simulink model "pitch_loop"  (Simulink 9.1)
settings: Solver=VariableStepAuto  StartTime=0.0  StopTime=10  RelTol=1e-3
values from neighbouring files (symbols this model uses):
  G = P.G    [getTF.m]
libraries: cstblocks x1
settings Model: LogicAnalyzerSignalOrdering=e66c3e0b-e53f-4c76-9941-291a87f7b6fd,76aed07c-1e48-440e-8e95-e8f535cd91f0,cd2aeb39-80bf-4c24-8e01-c28722cb3c59  Creator=leonardopedroso  LastModifiedBy=João Pinto
settings DataIOCC: SaveFormat=Dataset
settings OptimizationCC: LifeSpan=auto
settings DebuggingCC: UnderspecifiedInitializationDetection=Simplified  MergeDetectMultiDrivingBlocksExec=error  SFUnexpectedBacktrackingDiag=error  SFNoUnconditionalDefaultTransitionDiag=error  SFExecutionAtInitializationDiag=warning
settings HardwareCC: ProdBitPerPointer=64  ProdBitPerSizeT=64  ProdBitPerPtrDiffT=64  ProdLargestAtomicFloat=Float  ProdIntDivRoundTo=Zero  ProdEndianess=LittleEndian  ProdWordSize=64  ProdHWDeviceType=Intel->x86-64 (Windows64)
settings ModelReferenceCC: PropagateSignalLabelsOutOfModel=on
settings CodeAppCC: StateflowObjectComments=off
settings GRTTargetCC: TargetLangStandard=C99 (ISO)  CombineOutputUpdateFcns=on  GRTInterface=off
settings ConfigComp: CovMetricSettings=dwe  CovHtmlReporting=off  CovSaveCumulativeToWorkspaceVar=off  CovSaveSingleToWorkspaceVar=off  CovExternalEMLEnable=on

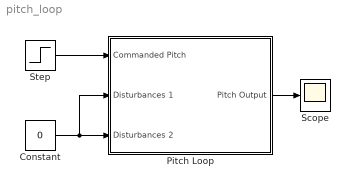
== system pitch_loop ==
  Constant : Constant  Value=0
  "Pitch Loop " : Subsystem
  Scope : Scope
  Step : Step  After=pi/9  SampleTime=0
  wires:
  Constant/1 -> "Pitch Loop "/2(Disturbances 1), "Pitch Loop "/3("Disturbances 2 ")
  "Pitch Loop "/1(Pitch Output) -> Scope/1
  Step/1 -> "Pitch Loop "/1(Commanded Pitch)

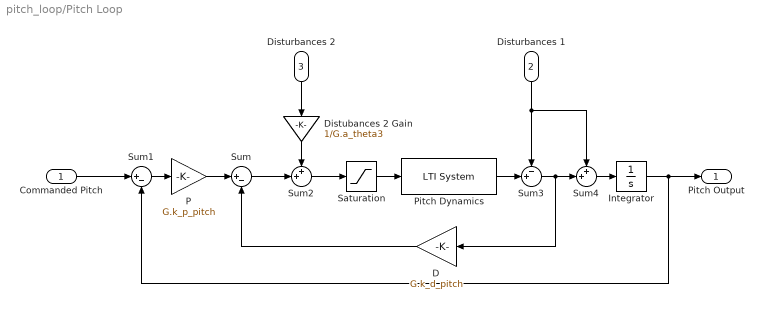
== system pitch_loop/Pitch Loop  ==
  Commanded Pitch : Inport
  Disturbances 1 : Inport  Port=2
  "Disturbances 2 " : Inport  Port=3
  D : Gain  Gain=G.k_d_pitch
  Distubances 2 Gain : Gain  Gain=1/G.a_theta3
  Integrator : Integrator
  "P " : Gain  Gain=G.k_p_pitch
  Pitch Dynamics : cstblocks/LTI System  sys=T_theta_dot_delta_e  IC=[]
  Saturation : Saturate  UpperLimit=G.delta_e_max  LowerLimit=-G.delta_a_max
  Sum : Sum  Inputs=|+-
  Sum1 : Sum  Inputs=|+-
  Sum2 : Sum  Inputs=++|
  Sum3 : Sum  Inputs=-+|
  Sum4 : Sum  Inputs=++|
  Pitch Output : Outport
  wires:
  Integrator/1 -> Pitch Output/1, Sum1/2
  Sum1/1 -> "P "/1
  Sum/1 -> Sum2/2
  Distubances 2 Gain/1 -> Sum2/1
  "Disturbances 2 "/1 -> Distubances 2 Gain/1
  Saturation/1 -> Pitch Dynamics/1
  "P "/1 -> Sum/1
  D/1 -> Sum/2
  Pitch Dynamics/1 -> Sum3/2
  Disturbances 1/1 -> Sum4/1, Sum3/1
  Sum3/1 -> D/1, Sum4/2
  Sum4/1 -> Integrator/1
  Sum2/1 -> Saturation/1
  Commanded Pitch/1 -> Sum1/1
